simulink model "slturtlesim"  (R2022a)
settings: Solver=FixedStepAuto  StartTime=0.0  StopTime=Inf  RelTol=1e-3
undefined symbols (not defined in the file): theta, x, y
libraries: ros2lib x3
settings Model: Creator=beave  LastModifiedBy=pi31415
settings OptimizationCC: EnhancedBackFolding=on  PassReuseOutputArgsAs=Individual arguments  ZeroExternalMemoryAtStartup=off  ZeroInternalMemoryAtStartup=off  MaxStackSize=64  OptimizeBlockOrder=speed  DifferentSizesBufferReuse=on  OptimizationCustomize=off  EfficientTunableParamExpr=on
settings DebuggingCC: ParameterTunabilityLossMsg=error  UnconnectedInputMsg=warning  UnconnectedOutputMsg=warning  UnconnectedLineMsg=warning
settings SFSimCC: MATLABDynamicMemAlloc=off
settings RTWCC: SystemTargetFile=ert.tlc  HardwareBoard=Robot Operating System 2 (ROS 2)  TemplateMakefile=ert_default_tmf  Toolchain=Colcon Tools  TargetLang=C++  DLArmComputeVersion=19.05
settings CodeAppCC: ForceParamTrailComments=on  IgnoreCustomStorageClasses=off  OperatorAnnotations=on  SimulinkDataObjDesc=on  SFDataObjDesc=on  InsertBlockDesc=on
settings ERTTargetCC: CodeInterfacePackaging=C++ class  SupportContinuousTime=on  RootIOFormat=Structure reference

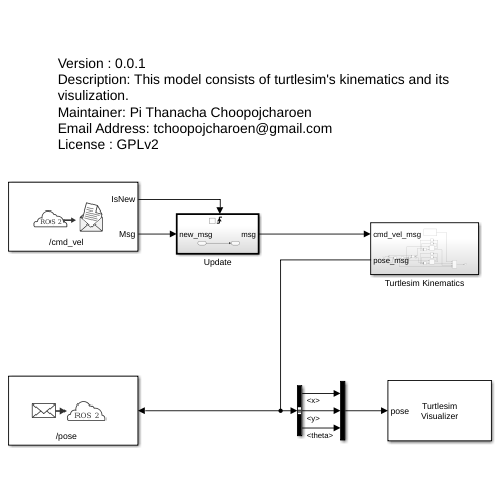
[thumbnail: Simulink's stored preview of the top-level diagram]
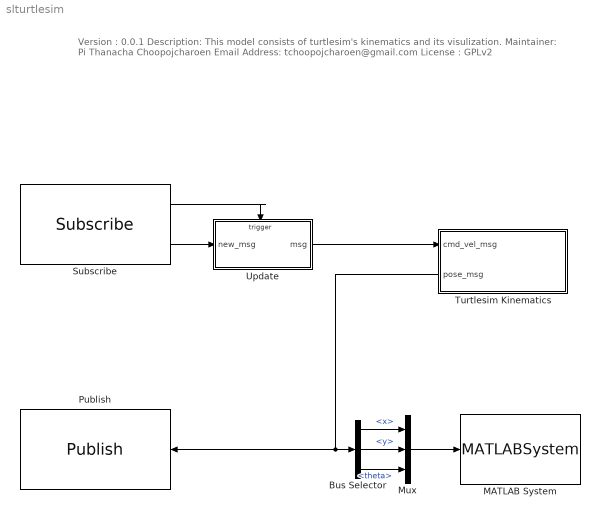
== system slturtlesim ==
  note: Version : 0.0.1
      | Description: This model consists of turtlesim's kinematics and its visulization.
      | Maintainer: Pi Thanacha Choopojcharoen
      | Email Address: tchoopojcharoen@gmail.com
      | License : GPLv2
  Bus Selector : BusSelector  OutputSignals=x,y,theta
  MATLAB System : MATLABSystem  System=TurtlesimVisualizer
      mask Type: TurtlesimVisualizer
      mask Display:
      | disp(['Turtlesim' char(10) 'Visualizer']);
      | port_label('input',1,'pose');
  Mux : Mux  Inputs=3
  Publish : ros2lib/Publish  topicSource=Specify your own  topic=/pose  messageType=turltlesim/Pose  QOSHistory=Keep last  QOSDepth=1  QOSReliability=Reliable  QOSDurability=Volatile
      settings: SourceProductBaseCode=RR
  Subscribe : ros2lib/Subscribe  topicSource=Specify your own  topic=/cmd_vel  messageType=geometry_msgs/Twist  sampleTime=-1  QOSHistory=Keep last  QOSDepth=1  QOSReliability=Reliable  QOSDurability=Volatile
      settings: SourceProductBaseCode=RR
  Turtlesim Kinematics : Subsystem
      settings: PortSchema="{\"entries\":[{\"content\":{\"sides\":[{\"content\":{\"connectorIds\":[\"In1\",\"Out1\"]},\"type\":\"ConnectorPlacement.EquallySpacedRectSide\",\"uuid\":\"6cc3d191-8b41-43a3-8d7e-fbb38f5f3909\"},{\"content\":{\"connectorIds\":[],\"side\":\"RIGHT\"},\"type\":\"ConnectorPlacement.EquallySpacedRectSide\",\"uuid\":\"02a725d1-914e-48c3-8213-963338e78503\"},{\"content\":{\"connectorIds\":[],\"side\":\"TOP\"},\"type\":\"ConnectorPlacement.EquallySpacedRectSide\",\"uuid\":\"a9769afc-f0de-40ec-971f-b36fa9ae13e3\"}]},\"type\":\"ConnectorPlacement.EquallySpacedConnector\",\"uuid\":\"c85e1385-84c4-4576-8165-8301e6039802\"}],\"packageUris\":[\"http://schema.mathworks.com/mf0/Connector/R2020b\"],\"version\":\"1.0\"}"
  Update : Subsystem
  wires:
  Mux/1 -> MATLAB System/1
  Bus Selector/2 -> Mux/2  "<y>"
  Bus Selector/3 -> Mux/3  "<theta>"
  Bus Selector/1 -> Mux/1  "<x>"
  Turtlesim Kinematics/1(pose_msg) -> Publish/1, Bus Selector/1
  Subscribe/2 -> Update/1(new_msg)
  Update/1(msg) -> Turtlesim Kinematics/1(cmd_vel_msg)
  Subscribe/1 -> Update/Trigger

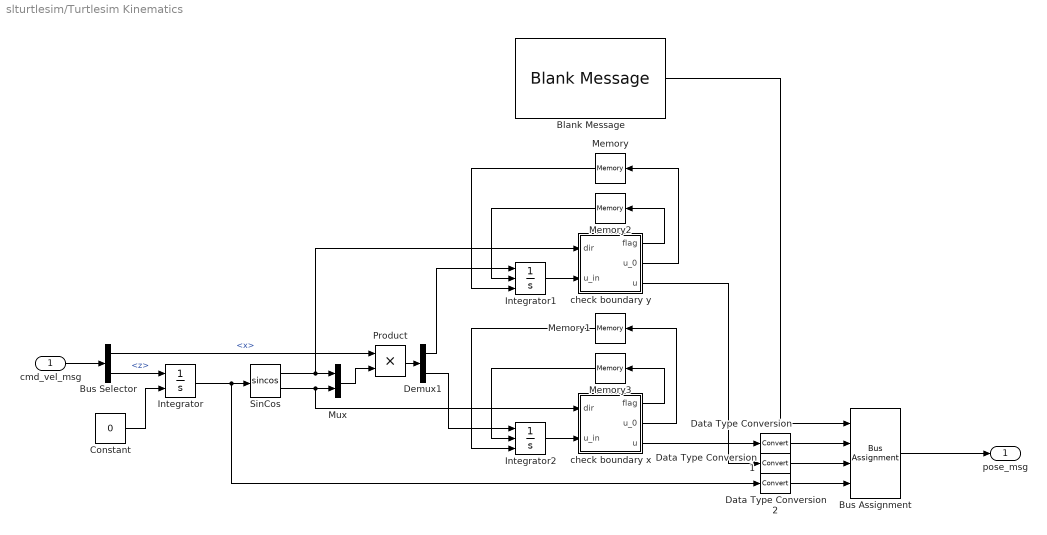
== system slturtlesim/Turtlesim Kinematics ==
  cmd_vel_msg : Inport  SampleTime=0.01
  Blank Message : ros2lib/Blank Message  messageClass=Message  entityType=turltlesim/Pose  messageType=turltlesim/Pose  SampleTime=inf
      settings: SourceProductBaseCode=RR
  Bus Assignment : BusAssignment  AssignedSignals=x,y,theta
  Bus Selector : BusSelector  OutputSignals=linear.x,angular.z
  Constant : Constant  Value=0
  Data Type Conversion : DataTypeConversion  SaturateOnIntegerOverflow=off  RndMeth=Floor
  Data Type Conversion1 : DataTypeConversion  SaturateOnIntegerOverflow=off  RndMeth=Floor
  Data Type Conversion2 : DataTypeConversion  SaturateOnIntegerOverflow=off  RndMeth=Floor
  Demux1 : Demux  Outputs=2
  Integrator : Integrator  InitialConditionSource=external
  Integrator1 : Integrator  ExternalReset=rising  InitialConditionSource=external
  Integrator2 : Integrator  ExternalReset=rising  InitialConditionSource=external
  Memory : Memory  InitialCondition=5
  Memory1 : Memory  InitialCondition=5
  Memory2 : Memory
  Memory3 : Memory
  Mux : Mux  Inputs=2
  Product : Product
  SinCos : Trigonometry  Operator=sincos
  check boundary x : Stateflow chart  TreatAsAtomicUnit=on
  check boundary y : Stateflow chart  TreatAsAtomicUnit=on
  pose_msg : Outport  SampleTime=0.01
  wires:
  Bus Assignment/1 -> pose_msg/1
  cmd_vel_msg/1 -> Bus Selector/1
  Mux/1 -> Product/2
  Blank Message/1 -> Bus Assignment/1
  Bus Selector/1 -> Product/1  "<x>"
  Bus Selector/2 -> Integrator/1  "<z>"
  Constant/1 -> Integrator/2
  Integrator/1 -> SinCos/1, Data Type Conversion2/1
  Product/1 -> Demux1/1
  Demux1/2 -> Integrator2/1
  SinCos/1 -> check boundary y/1(dir), Mux/1
  SinCos/2 -> check boundary x/1(dir), Mux/2
  Demux1/1 -> Integrator1/1
  Integrator1/1 -> check boundary y/2(u_in)
  Integrator2/1 -> check boundary x/2(u_in)
  check boundary y/1(flag) -> Memory2/1
  Memory2/1 -> Integrator1/2
  check boundary y/2(u_0) -> Memory/1
  Memory/1 -> Integrator1/3
  check boundary x/1(flag) -> Memory3/1
  Memory3/1 -> Integrator2/2
  check boundary x/2(u_0) -> Memory1/1
  Memory1/1 -> Integrator2/3
  check boundary y/3(u) -> Data Type Conversion1/1
  check boundary x/3(u) -> Data Type Conversion/1
  Data Type Conversion/1 -> Bus Assignment/2
  Data Type Conversion1/1 -> Bus Assignment/3
  Data Type Conversion2/1 -> Bus Assignment/4

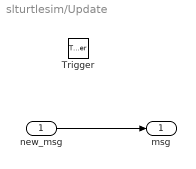
== system slturtlesim/Update ==
  new_msg : Inport
  Trigger : TriggerPort  VariantControl=(inherit)  PortDimensions=1
  msg : Outport
  wires:
  new_msg/1 -> msg/1

== stateflow chart slturtlesim/Turtlesim Kinematics/check boundary x ==
  state OutFieldLess
  state InField
    du:
    u = u_in;
  state OutFieldGreater
  (default) -> InField : {u=u_in;
      | flag = 1;
      | u_0 = 5;}
  InField -> OutFieldLess [order 1] : [(dir<0)&&(u<=0)]{u= 0;flag = 0;}
  InField -> OutFieldGreater [order 2] : [(dir>0)&&(u>=10)]{u= 10;flag = 0;}
  OutFieldGreater -> InField : [dir<=0]{u=u_in;flag = 1;u_0 = 10;}
  OutFieldLess -> InField : [dir>=0]{u=u_in;flag = 1;u_0 = 0;}
  data: flag output; u_0 output; dir input; u_in input; u output

== stateflow chart slturtlesim/Turtlesim Kinematics/check boundary y ==
  state OutFieldLess
  state InField
    du:
    u = u_in;
  state OutFieldGreater
  (default) -> InField : {u=u_in;
      | flag = 1;
      | u_0 = 5;}
  InField -> OutFieldLess [order 1] : [(dir<0)&&(u<=0)]{u= 0;flag = 0;}
  InField -> OutFieldGreater [order 2] : [(dir>0)&&(u>=10)]{u= 10;flag = 0;}
  OutFieldGreater -> InField : [dir<=0]{u=u_in;flag = 1;u_0 = 10;}
  OutFieldLess -> InField : [dir>=0]{u=u_in;flag = 1;u_0 = 0;}
  data: flag output; u_0 output; dir input; u_in input; u output
